simulink model "dyn_ext_sim"  (R2015b)
settings: Solver=ode1  StartTime=0.0  StopTime=20  FixedStep=0.002  MaxStep=0.1
settings Model: ExtModeTrigDuration=5000  Creator=robertph  LastModifiedBy=robertph
settings SolverCC: ZeroCrossControl=DisableAll  PositivePriorityOrder=on
settings RTWCC: SystemTargetFile=quarc_win64.tlc  TemplateMakefile=quarc_default_tmf  Description=QUARC Win64 Target
settings STFCustomTargetCC: GeneratePreprocessorConditionals=Use local settings  CPPClassGenCompliant=off
settings GRTTargetCC: ParMdlRefBuildCompliant=off  CompOptLevelCompliant=off  CombineOutputUpdateFcns=off  MatFileLogging=off  CPPClassGenCompliant=off  GRTInterface=on  UseToolchainInfoCompliant=off  ExtMode=on  ExtModeMexFile=quarc_comm

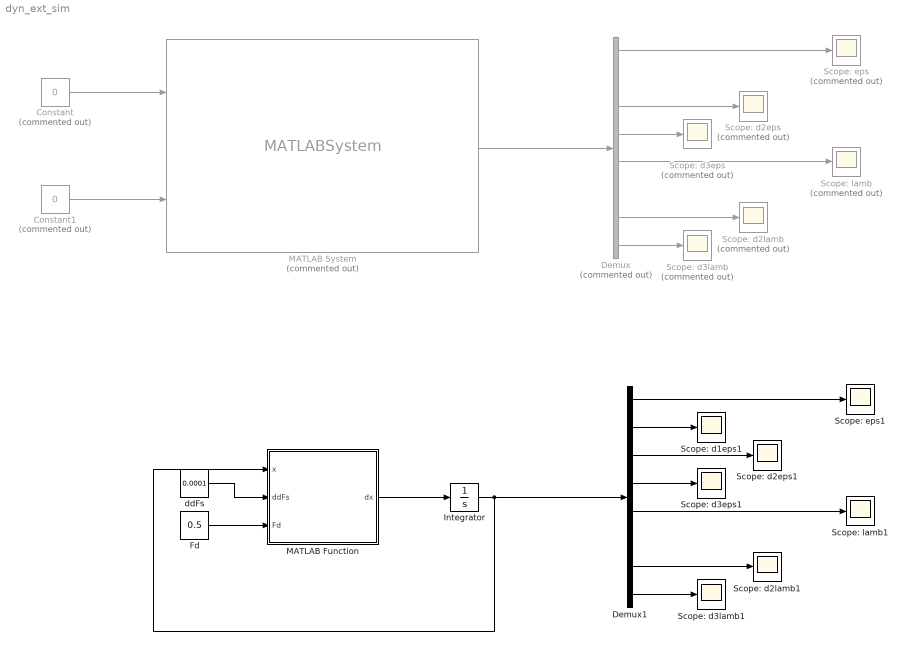
== system dyn_ext_sim ==
  Constant : Constant  Commented=on  Value=0
  Constant1 : Constant  Commented=on  Value=0
  Demux : Demux  Commented=on  Outputs=8
  Demux1 : Demux  Outputs=8
  Fd : Constant  Value=0.5
  Integrator : Integrator
  MATLAB Function : MATLAB Function  TreatAsAtomicUnit=on
  MATLAB System : MATLABSystem  Commented=on  System=DynamicExtensionSim  x0=zeros( 8, 1 )  step_width=0.002  SimulateUsing=Code generation
      mask Type: DynamicExtensionSim
      mask Display:
      | disp('DynamicExtensionSim');
      | port_label('input',1,'ddFs');
      | port_label('input',2,'Fd');
      | port_label('output',1,'x');
  Scope: d1eps1 : Scope
  Scope: d2eps : Scope  Commented=on
  Scope: d2eps1 : Scope
  Scope: d2lamb : Scope  Commented=on
  Scope: d2lamb1 : Scope
  Scope: d3eps : Scope  Commented=on
  Scope: d3eps1 : Scope
  Scope: d3lamb : Scope  Commented=on
  Scope: d3lamb1 : Scope
  Scope: eps : Scope  Commented=on
  Scope: eps1 : Scope
  Scope: lamb : Scope  Commented=on
  Scope: lamb1 : Scope
  ddFs : Constant  Value=0.0001
  wires:
  Constant/1 -> MATLAB System/1
  Constant1/1 -> MATLAB System/2
  MATLAB System/1 -> Demux/1
  Demux/1 -> Scope: eps/1
  Demux/5 -> Scope: lamb/1
  Demux/4 -> Scope: d3eps/1
  Demux/8 -> Scope: d3lamb/1
  Demux/3 -> Scope: d2eps/1
  Demux/7 -> Scope: d2lamb/1
  MATLAB Function/1(dx) -> Integrator/1
  Integrator/1 -> Demux1/1, MATLAB Function/1(x)
  Demux1/1 -> Scope: eps1/1
  Demux1/5 -> Scope: lamb1/1
  Demux1/4 -> Scope: d3eps1/1
  Demux1/8 -> Scope: d3lamb1/1
  Demux1/3 -> Scope: d2eps1/1
  Demux1/7 -> Scope: d2lamb1/1
  Fd/1 -> MATLAB Function/3(Fd)
  ddFs/1 -> MATLAB Function/2(ddFs)
  Demux1/2 -> Scope: d1eps1/1

== matlab function dyn_ext_sim/MATLAB Function ==
  data: x input; dx output; ddFs input; Fd input
function dx = fcn(x, ddFs, Fd)
%#codegen
persistent is_setup

if isempty(is_setup)
    is_setup = false;
end

if ~is_setup
    if coder.target('MATLAB')
        c_buildTapes_mex();
    else
        c_buildTapes();
    end
    
    is_setup = true;
end

if coder.target('MATLAB')
    gamma = c_calcGamma_mex(x);
    lambda = c_calcLambda_mex(x);
else
    gamma = c_calcGamma(x);
    lambda = c_calcLambda(x);
end

dx = zeros(8, 1);
u = [ddFs; Fd];

dx(1) = x(2);
dx(2) = x(3);
dx(3) = x(4);

dx(5) = x(6);
dx(6) = x(7);
dx(7) = x(8);

dx([4,8]) = gamma + lambda * u;
